simulink model "chienSearch_test_2020"  (R2020b)
settings: Solver=VariableStepAuto  StartTime=0.0  StopTime=10.0  RelTol=1e-3
settings Model: Creator=Jackie Smedley  LastModifiedBy=Dona
settings DebuggingCC: SFMachineParentedDataDiag=error

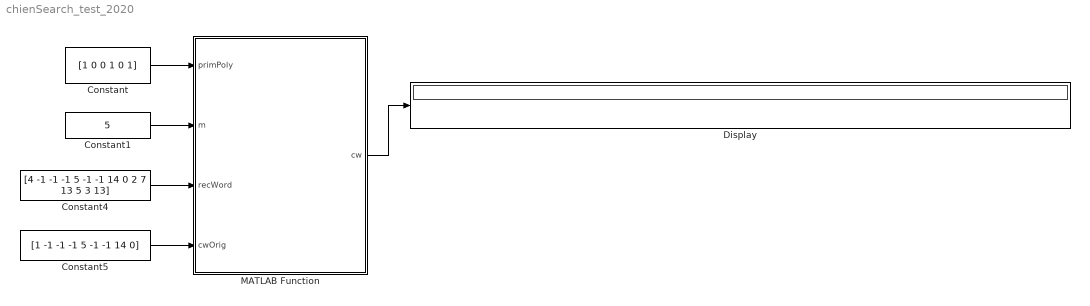
== system chienSearch_test_2020 ==
  Constant : Constant  Value=[1 0 0 1 0 1]  VectorParams1D=off
  Constant1 : Constant  Value=5
  Constant4 : Constant  Value=[4 -1 -1 -1 5 -1 -1 14 0 2 7 13 5 3 13]  VectorParams1D=off
  Constant5 : Constant  Value=[1 -1 -1 -1 5 -1 -1 14 0]  VectorParams1D=off
  Display : Display
  MATLAB Function : MATLAB Function  TreatAsAtomicUnit=on
  wires:
  MATLAB Function/1(cw) -> Display/1
  Constant1/1 -> MATLAB Function/2(m)
  Constant/1 -> MATLAB Function/1(primPoly)
  Constant4/1 -> MATLAB Function/3(recWord)
  Constant5/1 -> MATLAB Function/4(cwOrig)

== matlab function chienSearch_test_2020/MATLAB Function ==
  data: cw output; primPoly input; m input; recWord input; cwOrig input
function cw = fcn(primPoly, m, recWord, cwOrig)

    gf = GenerateGF2m(primPoly, int8(m));
    
    cw = ones(1, numel(recWord));
    temp_cw = BerlekampMasseyRS(recWord, gf, cwOrig);
    
    if temp_cw ~= -2
        for i = 1:numel(recWord)
            cw(i) = temp_cw(i); 
        end
    else
        for i = 1:numel(recWord)
            cw(i) = temp_cw; 
        end
    end
end
